simulink model "cart_pole_model"  (R2020b)
settings: Solver=VariableStepAuto  StartTime=0.0  StopTime=10.0  RelTol=1e-3
undefined symbols (not defined in the file): l, m
settings Model: Creator=Illia  LastModifiedBy=Illia

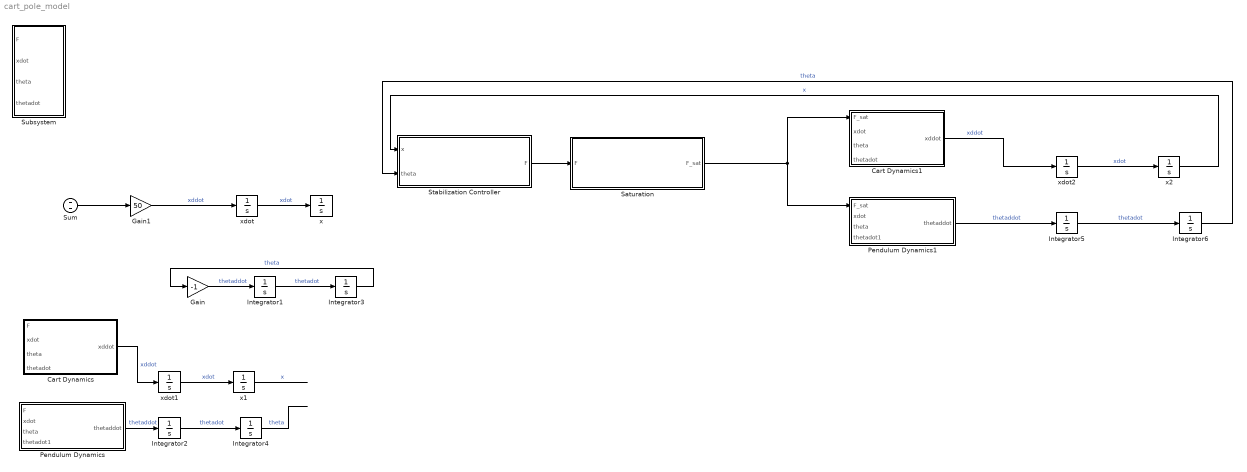
== system cart_pole_model ==
  Cart Dynamics : Subsystem
  Cart Dynamics1 : Subsystem
  Gain : Gain  Gain=-1
  Gain1 : Gain  Gain=50
  Integrator{1..6} (6 alike) : Integrator
  Pendulum Dynamics : Subsystem
  Pendulum Dynamics1 : Subsystem
  Saturation : Subsystem
  Stabilization Controller : Subsystem
  Subsystem : Subsystem
  Sum : Sum  Inputs=--
  x : Integrator
  x1 : Integrator
  x2 : Integrator
  xdot : Integrator
  xdot1 : Integrator
  xdot2 : Integrator
  wires:
  xdot/1 -> x/1  "xdot"
  Gain/1 -> Integrator1/1  "thetaddot"
  Integrator1/1 -> Integrator3/1  "thetadot"
  ? -> Sum/2  "theta"
  ? -> Sum/1  "x"
  Sum/1 -> Gain1/1
  Gain1/1 -> xdot/1  "xddot"
  Integrator3/1 -> Gain/1  "theta"
  Stabilization Controller/1(F) -> Saturation/1(F)
  Saturation/1(F_sat) -> Cart Dynamics1/1(F_sat), Pendulum Dynamics1/1(F_sat)
  Pendulum Dynamics1/1(thetaddot) -> Integrator5/1  "thetaddot"
  xdot2/1 -> x2/1  "xdot"
  Cart Dynamics1/1(xddot) -> xdot2/1  "xddot"
  Pendulum Dynamics/1(thetaddot) -> Integrator2/1  "thetaddot"
  Integrator2/1 -> Integrator4/1  "thetadot"
  Integrator4/1 -> ?  "theta"
  x1/1 -> ?  "x"
  xdot1/1 -> x1/1  "xdot"
  Cart Dynamics/1(xddot) -> xdot1/1  "xddot"
  Integrator5/1 -> Integrator6/1  "thetadot"
  Integrator6/1 -> Stabilization Controller/2(theta)  "theta"
  x2/1 -> Stabilization Controller/1(x)  "x"

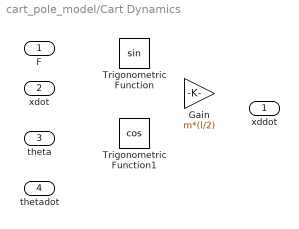
== system cart_pole_model/Cart Dynamics ==
  F : Inport
  xdot : Inport  Port=2
  theta : Inport  Port=3
  thetadot : Inport  Port=4
  Gain : Gain  Gain=m*(l/2)
  Trigonometric Function : Trigonometry
  Trigonometric Function1 : Trigonometry  Operator=cos
  xddot : Outport

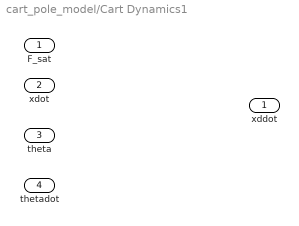
== system cart_pole_model/Cart Dynamics1 ==
  F_sat : Inport
  xdot : Inport  Port=2
  theta : Inport  Port=3
  thetadot : Inport  Port=4
  xddot : Outport

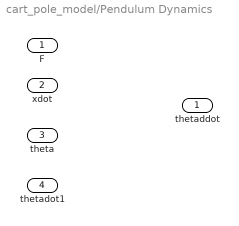
== system cart_pole_model/Pendulum Dynamics ==
  F : Inport
  xdot : Inport  Port=2
  theta : Inport  Port=3
  thetadot1 : Inport  Port=4
  thetaddot : Outport

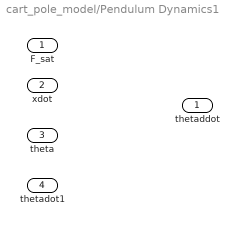
== system cart_pole_model/Pendulum Dynamics1 ==
  F_sat : Inport
  xdot : Inport  Port=2
  theta : Inport  Port=3
  thetadot1 : Inport  Port=4
  thetaddot : Outport

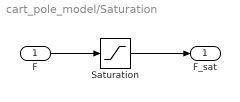
== system cart_pole_model/Saturation ==
  F : Inport
  Saturation : Saturate
  F_sat : Outport
  wires:
  F/1 -> Saturation/1
  Saturation/1 -> F_sat/1

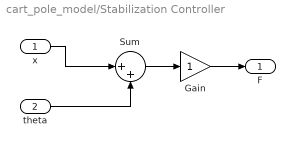
== system cart_pole_model/Stabilization Controller ==
  x : Inport
  theta : Inport  Port=2
  Gain : Gain
  Sum : Sum  Inputs=|++
  F : Outport
  wires:
  x/1 -> Sum/1
  theta/1 -> Sum/2
  Sum/1 -> Gain/1
  Gain/1 -> F/1

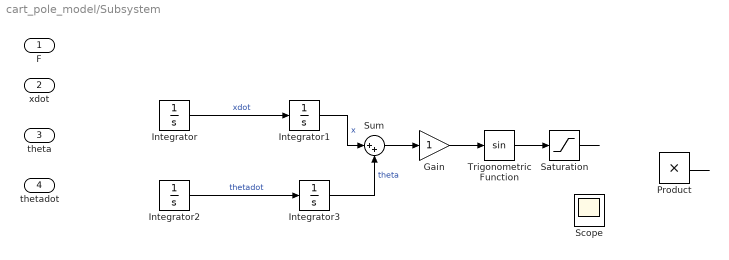
== system cart_pole_model/Subsystem ==
  F : Inport
  xdot : Inport  Port=2
  theta : Inport  Port=3
  thetadot : Inport  Port=4
  Gain : Gain
  Integrator{,1..3} (4 alike) : Integrator
  Product : Product
  Saturation : Saturate
  Scope : Scope
  Sum : Sum  Inputs=|++
  Trigonometric Function : Trigonometry
  wires:
  Trigonometric Function/1 -> Saturation/1
  Integrator/1 -> Integrator1/1  "xdot"
  Sum/1 -> Gain/1
  Integrator2/1 -> Integrator3/1  "thetadot"
  Saturation/1 -> ?
  Gain/1 -> Trigonometric Function/1
  Integrator3/1 -> Sum/2  "theta"
  Integrator1/1 -> Sum/1  "x"
  Product/1 -> ?
  ? -> Scope/1
  ? -> Integrator/1  "xddot"
  ? -> Integrator2/1  "thetaddot"
